simulink model "openloopPH"  (R2021a)
settings: Solver=VariableStepAuto  StartTime=0.0  StopTime=10.0  RelTol=1e-3
settings Model: Creator=USER  LastModifiedBy=USER

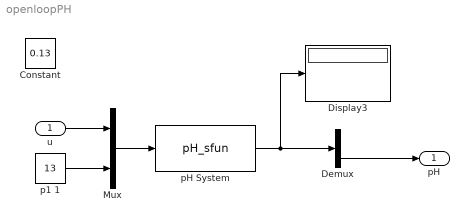
== system openloopPH ==
  u : Inport
  " p1 1" : Constant  Value=13
  Constant : Constant  Value=0.13
  Demux : Demux  Outputs=2
  Display3 : Display
  Mux : Mux  Inputs=2
  pH System : S-Function  FunctionName=pH_sfun  SFunctionDeploymentMode=off  EnableBusSupport=off
  pH : Outport
  wires:
  " p1 1"/1 -> Mux/2
  pH System/1 -> Demux/1, Display3/1
  u/1 -> Mux/1
  Mux/1 -> pH System/1
  Demux/2 -> pH/1
